simulink model "state_feedback"  (Simulink 6.6)
settings: Solver=ode5  StartTime=0.0  StopTime=50  FixedStep=0.001  RelTol=1e-3
InitFcn:
  | init_c
values from neighbouring files (symbols this model uses):
  j = [-1+sqrt(3)*i 0 0 0 0;0 -1-sqrt(3)*i 0 0 0; 0 0 -5 0 0; 0 0 0 -5 0; 0 0 0 0 -5 ]    [refrenceinputt.m]
undefined symbols (not defined in the file or in its folder): a, dzcv, fc, fp, fs, g, l, mi, xc, yc
settings Model: Creator=AF1  LastModifiedBy=AF1
settings DataIOCC: SignalLoggingName=sigsOut
settings OptimizationCC: BooleanDataType=off
settings DebuggingCC: SignalResolutionControl=TryResolveAllWithWarning  SolverPrmCheckMsg=none  MultiTaskDSMMsg=warning  MultiTaskCondExecSysMsg=none  StrictBusMsg=None
settings HardwareCC: TargetUnknown=on
settings RTWCC: IncludeERTFirstTime=on

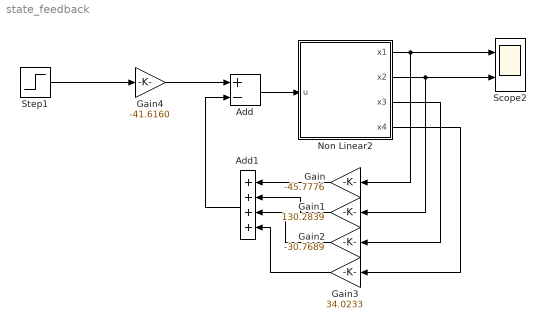
== system state_feedback ==
  Add : Sum  Inputs=+-  OutScaling=2^-10
  Add1 : Sum  Orientation=left  Inputs=++++  OutScaling=2^-10
  Gain : Gain  Orientation=left  Gain=-45.7776
  Gain1 : Gain  Orientation=left  Gain=130.2839
  Gain2 : Gain  Orientation=left  Gain=-30.7689
  Gain3 : Gain  Orientation=left  Gain=34.0233
  Gain4 : Gain  Gain=-41.6160
  Non Linear2 : Subsystem
  Scope2 : Scope  NumInputPorts=2
      settings: TimeRange=50  YMin=-0.04~-0.05  YMax=0.12~0.03999999999999999  SaveName=ScopeData2
  Step1 : Step  After=0.1  SampleTime=0
  wires:
  Add/1 -> Non Linear2/1(u)
  Non Linear2/1(x1) -> Scope2/1, Gain/1
  Non Linear2/2(x2) -> Scope2/2, Gain1/1
  Add1/1 -> Add/2
  Gain/1 -> Add1/1
  Gain1/1 -> Add1/2
  Gain2/1 -> Add1/3
  Gain3/1 -> Add1/4
  Non Linear2/3(x3) -> Gain2/1
  Non Linear2/4(x4) -> Gain3/1
  Step1/1 -> Gain4/1
  Gain4/1 -> Add/1

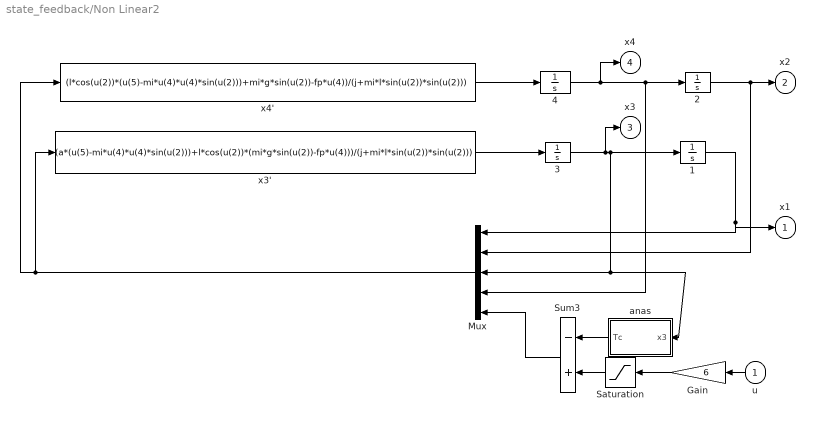
== system state_feedback/Non Linear2 ==
  u : Inport  Orientation=left
  1 : Integrator  InitialCondition=0.1
  2 : Integrator
  3 : Integrator
  4 : Integrator
  Gain : Gain  Orientation=left  Gain=6  SaturateOnIntegerOverflow=on
  Mux : Mux  Orientation=left  Inputs=5
  Saturation : Saturate  Orientation=left  UpperLimit=17  LowerLimit=-17
  Sum3 : Sum  Orientation=left  Inputs=-+  SaturateOnIntegerOverflow=on
  anas : Subsystem  Orientation=left
  x3' : Fcn  Expr=(a*(u(5)-mi*u(4)*u(4)*sin(u(2)))+l*cos(u(2))*(mi*g*sin(u(2))-fp*u(4)))/(j+mi*l*sin(u(2))*sin(u(2)))
  x4' : Fcn  Expr=(l*cos(u(2))*(u(5)-mi*u(4)*u(4)*sin(u(2)))+mi*g*sin(u(2))-fp*u(4))/(j+mi*l*sin(u(2))*sin(u(2)))
  x1 : Outport
  x2 : Outport  Port=2
  x3 : Outport  Port=3
  x4 : Outport  Port=4
  wires:
  4/1 -> 2/1, Mux/4, x4/1
  1/1 -> Mux/1, x1/1
  Mux/1 -> x4'/1, x3'/1
  u/1 -> Gain/1
  3/1 -> 1/1, Mux/3, anas/1(x3), x3/1
  2/1 -> Mux/2, x2/1
  Gain/1 -> Saturation/1
  anas/1(Tc) -> Sum3/1
  Sum3/1 -> Mux/5
  x4'/1 -> 4/1
  x3'/1 -> 3/1
  Saturation/1 -> Sum3/2

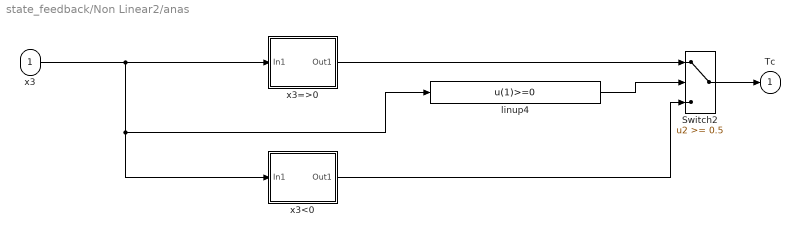
== system state_feedback/Non Linear2/anas ==
  x3 : Inport
  Switch2 : Switch  Threshold=0.5  SaturateOnIntegerOverflow=on
  linup4 : Fcn  Expr=u(1)>=0
  x3<0 : Subsystem
  x3=>0 : Subsystem
  Tc : Outport  OutDataType=fixdt(1,16,0)  OutScaling=[]
  wires:
  x3=>0/1(Out1) -> Switch2/1
  x3/1 -> x3=>0/1(In1), x3<0/1(In1), linup4/1
  x3<0/1(Out1) -> Switch2/3
  Switch2/1 -> Tc/1
  linup4/1 -> Switch2/2

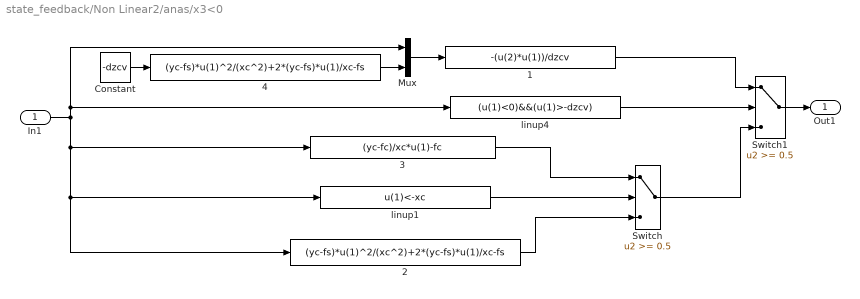
== system state_feedback/Non Linear2/anas/x3<0 ==
  In1 : Inport
  1 : Fcn  Expr=-(u(2)*u(1))/dzcv
  2 : Fcn  Expr=(yc-fs)*u(1)^2/(xc^2)+2*(yc-fs)*u(1)/xc-fs
  3 : Fcn  Expr=(yc-fc)/xc*u(1)-fc
  4 : Fcn  Expr=(yc-fs)*u(1)^2/(xc^2)+2*(yc-fs)*u(1)/xc-fs
  Constant : Constant  Value=-dzcv
  Mux : Mux  Inputs=2
  Switch : Switch  Threshold=0.5  SaturateOnIntegerOverflow=on
  Switch1 : Switch  Threshold=0.5  SaturateOnIntegerOverflow=on
  linup1 : Fcn  Expr=u(1)<-xc
  linup4 : Fcn  Expr=(u(1)<0)&&(u(1)>-dzcv)
  Out1 : Outport
  wires:
  Switch1/1 -> Out1/1
  In1/1 -> 2/1, linup1/1, 3/1, linup4/1, Mux/1
  Switch/1 -> Switch1/3
  linup1/1 -> Switch/2
  linup4/1 -> Switch1/2
  1/1 -> Switch1/1
  2/1 -> Switch/3
  3/1 -> Switch/1
  Mux/1 -> 1/1
  4/1 -> Mux/2
  Constant/1 -> 4/1

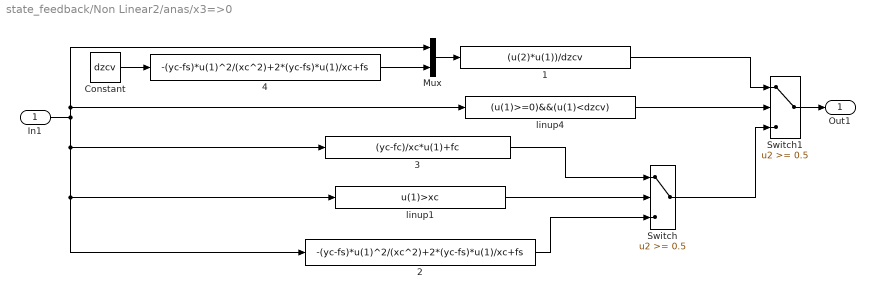
== system state_feedback/Non Linear2/anas/x3=>0 ==
  In1 : Inport
  1 : Fcn  Expr=(u(2)*u(1))/dzcv
  2 : Fcn  Expr=-(yc-fs)*u(1)^2/(xc^2)+2*(yc-fs)*u(1)/xc+fs
  3 : Fcn  Expr=(yc-fc)/xc*u(1)+fc
  4 : Fcn  Expr=-(yc-fs)*u(1)^2/(xc^2)+2*(yc-fs)*u(1)/xc+fs
  Constant : Constant  Value=dzcv
  Mux : Mux  Inputs=2
  Switch : Switch  Threshold=0.5  SaturateOnIntegerOverflow=on
  Switch1 : Switch  Threshold=0.5  SaturateOnIntegerOverflow=on
  linup1 : Fcn  Expr=u(1)>xc
  linup4 : Fcn  Expr=(u(1)>=0)&&(u(1)<dzcv)
  Out1 : Outport
  wires:
  3/1 -> Switch/1
  2/1 -> Switch/3
  1/1 -> Switch1/1
  linup4/1 -> Switch1/2
  linup1/1 -> Switch/2
  Switch/1 -> Switch1/3
  In1/1 -> 3/1, linup1/1, 2/1, linup4/1, Mux/1
  Switch1/1 -> Out1/1
  Mux/1 -> 1/1
  4/1 -> Mux/2
  Constant/1 -> 4/1
